simulink model "Fzgsym_MtrSpdxx"  (R2022b)
settings: Solver=VariableStepAuto  StartTime=0.0  StopTime=1830  RelTol=1e-3
values from neighbouring files (symbols this model uses):
  g = 9.81    [Energiebedarf_single.m]
  m = 1500    [Energiebedarf_single.m]
undefined symbols (not defined in the file or in its folder): air_temp, battPwrChrgLmt, battPwrDischrgLmt, brkpoints_Lmt, brkprs_front, brkprs_max, brkprs_rear, disk_abore, efficiency, l_CG_rear, mass_veh, mu_kinetic, nmo_rpm, num_mot, num_p, num_pads, r_m, speedEff_rpm, trq, trq_eff
libraries: autolibshared x8, simulink x7, autolibmappedmotor x4, autolibutils x1, autolibdatasheetbattery x1
(part 1 of 4)
settings Model: Creator=ferdi  LastModifiedBy=ferdi
settings ModelReferenceCC: EnableRefExpFcnMdlSchedulingChecks=on

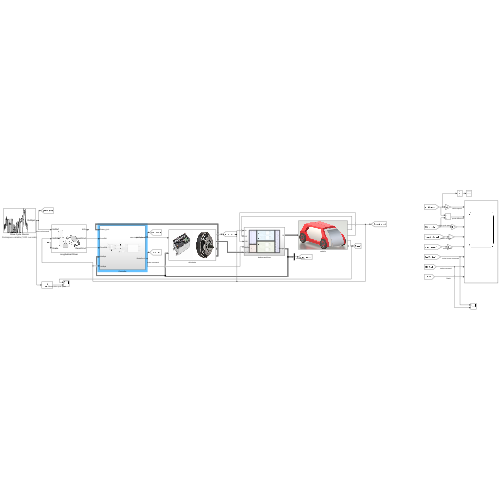
[thumbnail: Simulink's stored preview of the top-level diagram]
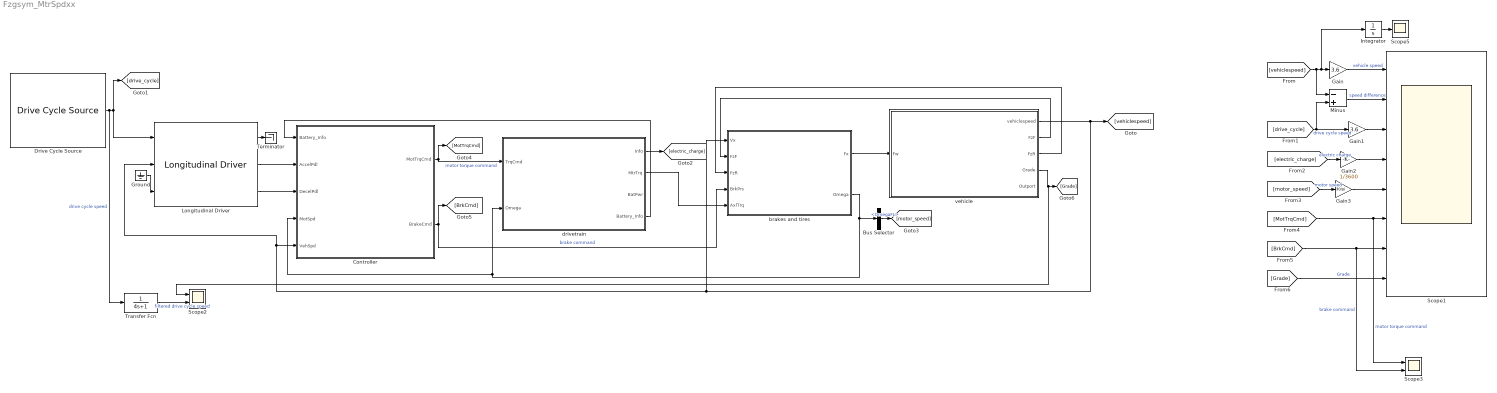
== system Fzgsym_MtrSpdxx ==
  Bus Selector : BusSelector  OutputSignals=OmegaFL
  Controller : Subsystem
  Drive Cycle Source : autolibshared/Drive Cycle Source  cycleVar=Workspace variable  wsVar=myCycle  fileVar=C:\Users\ferdi\OneDrive\Dokumente\MATLAB\Hiwi\HElmar\Strecke.mat  tfinal="1830  seconds"  cycleRepeat=off  outAccPort=off  outGearPort=off  gearList=No gear data  t_wot1=5  xdot_woto=0  xdot_wot1=3  t_wot2=45  xdot_wot2=0  t_wotend=50  srcUnit=m/s  outUnit=m/s  srcAccUnit=m/s/s  outAccUnit=m/s^2  dt=0  aMode=1  faultOption=off  velBnd=2  velBndUnit=mph  inUnit=m/s  timeBnd=1  failOption=off  stopSim=off  maxFaultCnt=10  maxFaultTime=2  maxTotFaultTime=15  traceOption=off  dtTrace=1  traceWindow=10  lastDCname=Custom Data Set  lastOutUnit=mph  lastDT=0  lastTB=1  lastSB=2  forceCalcBound=off
  Gain : Gain  Gain=3.6
  Gain1 : Gain  Gain=3.6
  Gain2 : Gain  Gain=1/3600
  Gain3 : Gain  Gain=30/pi
  Ground : Ground
  Integrator : Integrator
  Longitudinal Driver : autolibshared/Longitudinal Driver  extAccelOvr=off  extDecelOvr=off  extAccelHld=off  extDecelHld=off  extAccelZero=off  extDecelZero=off  cntrlType=PI  shftType=None  velUnits=m/s  gearOut=off  Kp=5  Ki=25  Kff=.05  Kg=0.01  VehVelVec=gain_velocity  KffVec=gain_velocity_ff  KpVec=gain_proportional  KiVec=gain_integral  KgVec=grade_angle_ff  m=780  Kpt=3000  tau=.1  L=10  aR=200  bR=2.5  cR=.5  g=9.81  vnom=v_nom  Kaw=kaw  tauerr=tauerr  tauPt=2  GearInit=0  tShift=.1  pdlVec=[0.1 0.4 0.5 0.9]  upShftTbl=[-1 12.9375 26.4375 39.9375 51.18749999999999 62.4375 72.84375 83.25;-1 16.3125 29.8125 43.3125 54.5624 65.8125 76.78125 87.75;-1 19.6875 33.1875 46.68749999999999 57.9375 69.1875 80.71875 92.25;-1 33 52.5 77.25 100.5 138.75 161.875 185]  dwnShftTbl=[1 9.5625 23.0625 36.5625 47.8125 59.0625 68.90625 78.75;1 12.9375 26.4375 39.9375 51.18749999999999 62.4375 72.84375 83.25;1 16.3125 29.8125 43.3125 54.562499 65.8125 76.78125 87.75;1 19.6875 33.1875 46.68749999999999 57.9375 69.1875 80.71875 92.25]  tClutch=.5  tRev=.5  tPark=120  aMode=1  UpGearVec="[0  1  2  3  4  5  6  7]"  DownGearVec="[1  2  3  4  5  6  7  8]"
  Minus : Sum  Inputs=-+
  Scope1 : Scope  NumInputPorts=8
  Scope2 : Scope  NumInputPorts=2
  Scope3 : Scope  NumInputPorts=2
  Scope5 : Scope
  Terminator : Terminator
  Transfer Fcn : TransferFcn  Denominator=[4 1]
  brakes and tires : Subsystem
  drivetrain : Subsystem
      mask Display: image('C:\Users\ferdi\OneDrive\Dokumente\MATLAB\Hiwi\HElmar\Bilder\Batterie_Motor.png'); % Use "Edit Image" on toolstrip to change.
  vehicle : Subsystem
      mask Display: image('C:\Users\ferdi\OneDrive\Dokumente\MATLAB\Hiwi\HElmar\Bilder\HEImar.png'); % Use "Edit Image" on toolstrip to change.
  wires:
  Drive Cycle Source/1 -> Transfer Fcn/1, Longitudinal Driver/1, [drive_cycle]  "drive cycle speed"
  Ground/1 -> Longitudinal Driver/3
  Longitudinal Driver/2 -> Controller/2(AccelPdl)
  Longitudinal Driver/3 -> Controller/3(DecelPdl)
  brakes and tires/2(Omega) -> Bus Selector/1, drivetrain/2(Omega), Controller/4(MotSpd)
  Controller/2(BrakeCmd) -> brakes and tires/4(BrkPrs), [BrkCmd]  "brake command"
  vehicle/1(vehiclespeed) -> Longitudinal Driver/2, Controller/5(VehSpd), brakes and tires/1(Vx), [vehiclespeed]
  vehicle/2(FzF) -> brakes and tires/2(FzF)
  vehicle/3(FzR) -> brakes and tires/3(FzR)
  Controller/1(MotTrqCmd) -> [MotTrqCmd], drivetrain/1(TrqCmd)  "motor torque command"
  Longitudinal Driver/1 -> Terminator/1
  brakes and tires/1(Fx) -> vehicle/1(Fw)
  drivetrain/2(MtrTrq) -> brakes and tires/5(AxlTrq)
  [vehiclespeed] -> Minus/1, Integrator/1, Gain/1
  [drive_cycle] -> Minus/2, Gain1/1  "drive cycle speed"
  drivetrain/1(Info) -> [electric_charge]
  [electric_charge] -> Gain2/1  "electric charge"
  Bus Selector/1 -> [motor_speed]  "<OmegaFL>"
  [motor_speed] -> Gain3/1  "motor speed"
  [BrkCmd] -> Scope3/2, Scope1/7  "brake command"
  [MotTrqCmd] -> Scope3/1, Scope1/6  "motor torque command"
  Gain/1 -> Scope1/1  "vehicle speed"
  Minus/1 -> Scope1/2  "speed difference"
  vehicle/4(Grade) -> Scope2/1, [Grade]
  [Grade] -> Scope1/8  "Grade"
  Transfer Fcn/1 -> Scope2/2  "filtered drive cycle speed"
  Gain1/1 -> Scope1/3
  Integrator/1 -> Scope5/1
  Gain2/1 -> Scope1/4
  Gain3/1 -> Scope1/5
  drivetrain/4(Battery_Info) -> Controller/1("Battery_Info ")

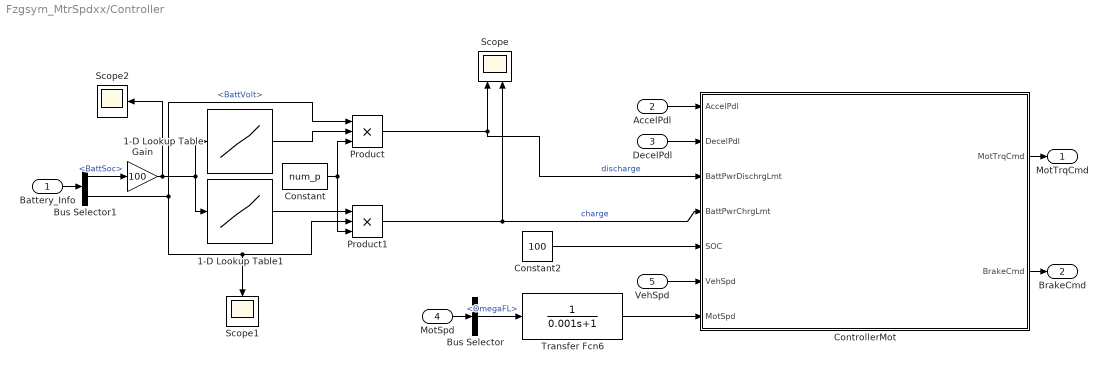
== system Fzgsym_MtrSpdxx/Controller ==
  "Battery_Info " : Inport
  AccelPdl : Inport  Port=2
  DecelPdl : Inport  Port=3
  MotSpd : Inport  Port=4
  VehSpd : Inport  Port=5
  1-D Lookup Table : Lookup_n-D  NumberOfTableDimensions=1  BreakpointsForDimension1=brkpoints_Lmt  Table=battPwrDischrgLmt  InternalRulePriority=Speed  RndMeth=Simplest
  1-D Lookup Table1 : Lookup_n-D  NumberOfTableDimensions=1  BreakpointsForDimension1=brkpoints_Lmt  Table=battPwrChrgLmt  InternalRulePriority=Speed  RndMeth=Simplest
  Bus Selector : BusSelector  OutputSignals=OmegaFL
  Bus Selector1 : BusSelector  OutputSignals=BattSoc,BattVolt
  Constant : Constant  Value=num_p
  Constant2 : Constant  Value=100
  ControllerMot : Subsystem
  Gain : Gain  Gain=100
  Product : Product  Inputs=3
  Product1 : Product  Inputs=3
  Scope : Scope  NumInputPorts=2
  Scope1 : Scope
  Scope2 : Scope
  Transfer Fcn6 : TransferFcn  Denominator=[0.001 1]
  MotTrqCmd : Outport
  BrakeCmd : Outport  Port=2
  wires:
  AccelPdl/1 -> ControllerMot/1(AccelPdl)
  VehSpd/1 -> ControllerMot/6(VehSpd)
  DecelPdl/1 -> ControllerMot/2(DecelPdl)
  ControllerMot/1(MotTrqCmd) -> MotTrqCmd/1
  ControllerMot/2(BrakeCmd) -> BrakeCmd/1
  Constant2/1 -> ControllerMot/5(SOC)
  Product1/1 -> Scope/2, ControllerMot/4(BattPwrChrgLmt)  "charge"
  Product/1 -> ControllerMot/3(BattPwrDischrgLmt), Scope/1  "discharge"
  MotSpd/1 -> Bus Selector/1
  Bus Selector/1 -> Transfer Fcn6/1  "<OmegaFL>"
  Transfer Fcn6/1 -> ControllerMot/7(MotSpd)
  Gain/1 -> 1-D Lookup Table/1, 1-D Lookup Table1/1, Scope2/1
  1-D Lookup Table/1 -> Product/2
  1-D Lookup Table1/1 -> Product1/1
  "Battery_Info "/1 -> Bus Selector1/1
  Bus Selector1/1 -> Gain/1  "<BattSoc>"
  Bus Selector1/2 -> Product/1, Scope1/1, Product1/2  "<BattVolt>"
  Constant/1 -> Product/3, Product1/3
